simulink model "fuelcell"  (R2023a)
settings: Solver=VariableStepAuto  StartTime=0.0  StopTime=20  RelTol=1e-3
model workspace (MAT data in the model file):
  sweep1 = [0 5 10 15 20 25 30 35 40 45 50 55 60 65 70 75 80]
libraries: fl_lib x24, nesl_utility x12, ee_lib x2, spsCurrentVoltageSimscapeInterfaceLib x1, spsFuelCellStackLib x1, sps_lib x1
settings Model: Creator=connl  LastModifiedBy=connl

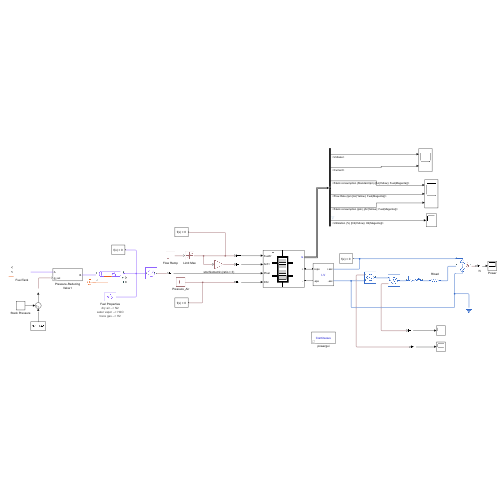
[thumbnail: Simulink's stored preview of the top-level diagram]
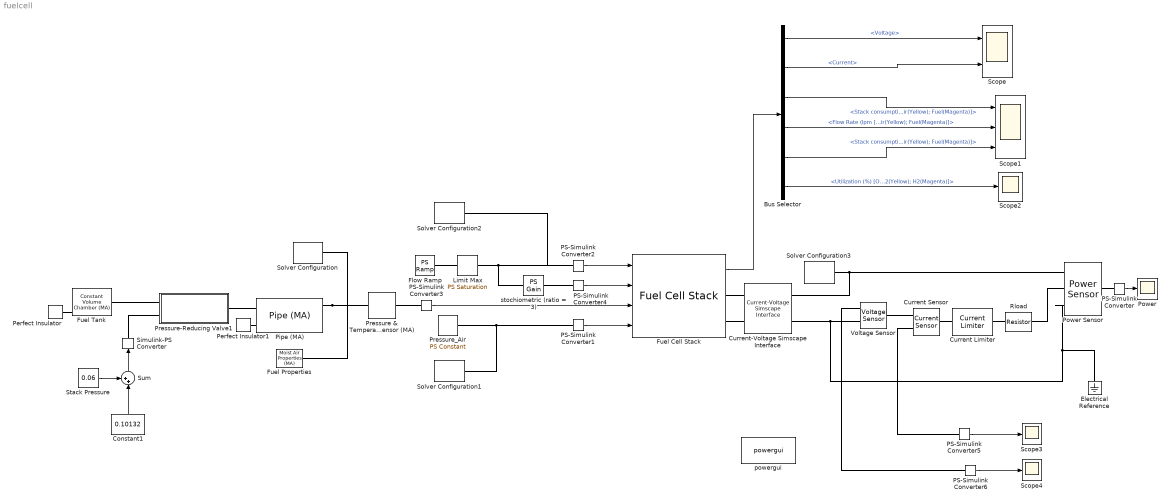
== system fuelcell ==
  Bus Selector : BusSelector  OutputSignals=Voltage,Current,Stack consumption (Standard lpm) [Air(Yellow); Fuel(Magenta)],Flow Rate (lpm [Air(Yellow); Fuel(Magenta)],Stack consumption (lpm) [Air(Yellow); Fuel(Magenta)],Utilization (%) [O2(Yellow); H2(Magenta)]
  Constant1 : Constant  Value=0.10132
  Current Limiter : ee_lib/Semiconductors & Converters/Current Limiter  iLim=80 A  vLim=0.1 V  gLim=1e-3 1/Ohm  thermal_mass=100 J/K  initial_temperature=298.15 K
      settings: InternalSimscapePortConfiguration="{\"Bottom\":[],\"Left\":[{\"id\":\"p\",\"label\":\"+\",\"type\":\"foundation.electrical.electrical\"}],\"Right\":[{\"id\":\"n\",\"label\":\"-\",\"type\":\"foundation.electrical.electrical\"}],\"Top\":[]}"
  Current Sensor : fl_lib/Electrical/Electrical Sensors/Current Sensor
  Current-Voltage Simscape Interface : spsCurrentVoltageSimscapeInterfaceLib/Current-Voltage Simscape Interface  DFT=off  FMode=Low pass filter (continuous)  T=1e-6  Ts=50e-6  i0=0  v0=0  Sd=Specialized Power Systems side  Measurements=off
      settings: LibrarySourceBlock=|
      | sps_lib/Utilities/Current-Voltage
      | Simscape Interface
  Electrical Reference : fl_lib/Electrical/Electrical Elements/Electrical Reference
  Flow Ramp : fl_lib/Physical Signals/Sources/PS Ramp  slope=1.667 lpm/s  start_time=0 s  initial_output=2 lpm
  Fuel Cell Stack : spsFuelCellStackLib/Fuel Cell Stack  PresetModel=PEMFC - 1.26 kW - 24 Vdc  FcType=0  Detailed=Detailed  Eoc=[42,35]  NomVI=[52,24.23]  EndVI=[100,20]  Nc=42  n=46  TOp=55  AirFr=2400  SuppPress=[1.5,1]  Comp=[99.95,21,1]  SignX=off  SignY=off  FlowRateH2=on  FlowRateAir=on  SystemTemp=off  SystemPH2=on  SystemPAir=on  FCDyn=off  FC_tau=1  Peak_O2=80  V_Under=10
      settings: LibrarySourceBlock=sps_lib/Sources/Fuel Cell Stack
  Fuel Properties : fl_lib/Moist Air/Utilities/Moist Air Properties (MA)  R_a=296.8 J/kg/K  T_TLU=[-56.55 -50 -40 -30 -20 -10 -5 -4 -3 -2 -1 0 1 2 3 4 5 10 20 30 40 50 60 70 80 90 100 110 120 130 140 150 160 170 180 190 200 210 220 230 240 250 260 270 280 290 300 310 320 330 340 350] degC  h_a_TLU=[224.312019475783 231.141016528663 241.564116974996 251.984329606098 262.402210767198 272.818266126753 278.025759131002 279.067222480148 280.108675169779 281.150117667373 282.191550440608 283.232973957487 284.274388686473 285.315795096618 286.357193657682 287.39858484026 288.439969115894 293.646803474573 304.06022922571 314.473742203777 324.887858161051 335.303123493654 345.720119003427 356.139461810715 366.561805672305 376.987839945795 387.418287430292 397.85390130103 408.295461341278 418.743769658649 429.199646054884 439.663923199077 450.137441734658 460.621045430963 471.115576471389 481.621870952319 492.140754650669 502.67303910305 513.219518026408 523.780964098585 534.358126107445 544.951726469054 555.562459108678 566.190987693008 576.837944197865 587.503927792527 598.189504019663 608.89520424844 619.621525377624 630.368929765337 641.137845362314 651.928666026144] kJ/kg  mu_a_TLU=[13.7948920665312 14.136718735151 14.6513506072199 15.1575394445859 15.6556177860831 16.1459023391225 16.3882166949119 16.4364580271216 16.484626183061 16.5327214469937 16.5807441017456 16.6286944287114 16.6765727078615 16.7243792177482 16.7721142355126 16.8197780368914 16.8673708962236 17.1042805670559 17.5729330929829 18.0349108462106 18.4904598524977 18.9398140034241 19.3831957199835 19.8208165930053 20.2528779961256 20.6795716689317 21.101080269236 21.5175778943589 21.9292305719283 22.3361967211248 22.7386275855675 23.1366676391963 23.5304549665897 23.9201216191847 24.3057939488592 24.6875929202991 25.0656344035241 25.4400294478834 25.8108845387614 26.178301838167 26.5423794103038 26.9032114331518 27.2608883970194 27.6154972909606 27.96712177789 28.315842359167 28.6617365293689 29.0048789219164 29.3453414461711 29.6831934165754 30.0185016743671 30.3513307023604] s*uPa  k_a_TLU=[19.6296532607374 20.1533289725195 20.9436243615696 21.7231523445233 22.492306313909 23.2514823266989 23.6274403302585 23.7023472871786 23.7771601872884 23.8518793809024 23.9265052168265 24.0010380423605 24.0754782033001 24.1498260439393 24.2240819070729 24.2982461339996 24.3723190645241 24.7413260601341 25.4726839899413 26.1954347636057 26.9098870600572 27.6163358040134 28.3150627088262 29.0063368423447 29.6904152006066 30.3675432785589 31.0379556302294 31.7018764131555 32.3595199136277 33.0110910505971 33.6567858570436 34.2967919382928 34.9312889072676 35.5604487970156 36.1844364511046 36.8034098926428 37.417520672793 38.0269141997105 38.63173004887 39.2321022557508 39.828159591842 40.4200258249072 41.0078199644172 41.591656493024 42.171645584909 42.7478933117983 43.3205018373934 43.8895696009277 44.4551914905138 45.0174590069098 45.5764604182929 46.1322809065919] mW/m/K  p_min=1 kPa  p_max=inf MPa  T_min=-56.55 degC  T_max=350 degC  properties_range_check=simscape.enum.assert.action.error  p_atm=0.101325 MPa  T_atm=20 degC  R_w=461.523 J/kg/K  p_ws_TLU=[1.71168953425982e-06; 3.93770601979424e-06; 1.28411717710344e-05; 3.80051394873809e-05; .00010323902900209; .000259873810798063; .000401741022116384; .000437454836117844; .000476040820618202; .000517704666185737; .000562664883741207; .000611212677444345; .000657088049117899; .000705987905898279; .000758082381149132; .000813549384183233; .000872574861129522; .00122818386934022; .0023392147667769; .00424668834054807; .00738442748706953; .0123512704340234; .0199458019246787; .0312006356960619; .0474147199263783; .0701823607447713; .10141797792131; .143375967241115; .198665399739302; .270259606559999; .361500961984849; .476101381081492; .618139196722055; .792053183687694; 1.0026345688121; 1.25501792086105; 1.55467186826983; 1.90739066433297; 2.31928772772542; 2.79679245576864; 3.34665187151016; 3.97593907083533; 4.69207105435535; 5.5028394740883; 6.41645928168037; 7.4416425436169; 8.58770832955728; 9.86474556030261; 11.2838558865497; 12.8575218898034; 14.6001810568052; 16.5291642526045] MPa  h_w_vap_TLU=[2836.88241275372; 2837.81392500514; 2838.63937175807; 2838.7309929628; 2838.06905313927; 2836.62597341095; 2835.60023952573; 2835.37006381376; 2835.13143158077; 2834.88429145066; 2834.62859062897; 2500.93420564316; 2498.55329907119; 2496.17495082036; 2493.79885912205; 2491.42474723191; 2489.05236104642; 2477.20875029194; 2453.54955988604; 2429.83856603313; 2406.00136954922; 2381.97406342174; 2357.69101156389; 2333.08088387814; 2308.06565480412; 2282.56034405021; 2256.47287422313; 2229.70428017508; 2202.14968030993; 2173.69998896199; 2144.24368406447; 2113.66758247452; 2081.85585110571; 2048.68725710494; 2014.03141249899; 1977.7449923284; 1939.66849592886; 1899.62342931686; 1857.40930169838; 1812.79975416601; 1765.53721731251; 1715.32525772152; 1661.81700477787; 1604.59703745016; 1543.1534616334; 1476.83692476464; 1404.80240352424; 1325.92091736114; 1238.61667822208; 1140.5102987018; 1027.62017777647; 892.733785613825] kJ/kg  h_w_TLU=[2396.55944251649; 2408.68643343608; 2427.1988031141; 2445.702165897; 2464.18429108356; 2482.62529466839; 2491.82135326629; 2493.6580151792; 2495.49372578218; 2497.32843835745; 2499.16210446923; 2500.99462758899; 2502.83092214066; 2504.6665223621; 2506.50140563013; 2508.335548891; 2510.16892865793; 2519.32352241995; 2537.56068088674; 2555.67742615292; 2573.6403223998; 2591.4109179101; 2608.9455037701; 2626.19492016262; 2643.10444358428; 2659.61377634497; 2675.58278696023; 2696.1846256545; 2716.49989553741; 2736.6235210957; 2756.61216047011; 2776.50561773853; 2796.33378922508; 2816.11979583049; 2835.88181423877; 2855.63430574511; 2875.38889327595; 2895.15500577172; 2914.94035964689; 2934.75132290228; 2954.59319330244; 2974.47041285505; 2994.38673458964; 3014.34535328009; 3034.34900867103; 3054.40006755764; 3074.50058946898; 3094.65237953784; 3114.85703128106; 3135.11596137801; 3155.43043805905; 3175.80160435813] kJ/kg  mu_w_TLU=[6.81365662228272; 7.04953750742707; 7.40970098298307; 7.76991278093907; 8.13017290129507; 8.49048134405107; 8.67065368632907; 8.70668960445667; 8.74272600580827; 8.77876289038387; 8.81480025818347; 8.85083810920707; 8.88687644345467; 8.92291526092627; 8.95895456162187; 8.99499434554147; 9.03103461268507; 9.21124319676307; 9.57169660671907; 9.93219833907507; 10.2927483938311; 10.6533467709871; 11.0139934705431; 11.3746884924991; 11.7354318368551; 12.0962235036111; 12.4570634927671; 12.8179518043231; 13.1788884382791; 13.5398733946351; 13.9009066733911; 14.2619882745471; 14.6231181981031; 14.9842964440591; 15.3455230124151; 15.7067979031711; 16.0681211163271; 16.4294926518831; 16.7909125098391; 17.1523806901951; 17.5138971929511; 17.8754620181071; 18.2370751656631; 18.5987366356191; 18.9604464279751; 19.3222045427311; 19.6840109798871; 20.0458657394431; 20.4077688213991; 20.7697202257551; 21.1317199525111; 21.4937680016671] s*uPa  k_w_TLU=[11.46288215976; 11.941997488935; 12.676358586935; 13.414208884935; 14.155548382935; 14.900377080935; 15.274099879935; 15.348949115735; 15.423833243535; 15.498752263335; 15.573706175135; 15.648694978935; 15.723718674735; 15.798777262535; 15.873870742335; 15.948999114135; 16.024162377935; 16.400502076935; 17.155798374935; 17.914583872935; 18.676858570935; 19.442622468935; 20.211875566935; 20.984617864935; 21.760849362935; 22.540570060935; 23.323779958935; 24.110479056935; 24.900667354935; 25.694344852935; 26.491511550935; 27.292167448935; 28.096312546935; 28.903946844935; 29.715070342935; 30.529683040935; 31.347784938935; 32.169376036935; 32.994456334935; 33.823025832935; 34.655084530935; 35.490632428935; 36.329669526935; 37.172195824935; 38.018211322935; 38.867716020935; 39.720709918935; 40.577193016935; 41.437165314935; 42.300626812935; 43.167577510935; 44.038017408935] mW/m/K  D_w=25 mm^2/s  trace_gas_model=foundation.enum.trace_gas_model.track_properties  R_g=4124.48151675695 J/kg/K  h_g_TLU=[2783.66044045879 2873.94181645932 3012.62601981068 3152.22537301871 3292.62486344326 3433.7213835968 3504.50184295996 3518.67512520997 3532.85394543712 3547.03822323045 3561.22787913325 3575.42283463482 3589.62301216223 3603.82833507219 3618.0387276429 3632.25411506595 3646.4744234383 3717.64725530348 3860.3219873489 4003.3828816304 4146.77354613486 4290.44463593559 4434.35318483605 4578.46197843019 4722.7389683309 4867.15672726297 5011.69194456718 5156.32496143709 5301.03934494342 5445.82149962224 5590.6603151415 5735.54684833147 5880.47403768083 6025.43644826542 6170.4300449914 6315.45199199528 6460.50047604533 6605.57455182556 6750.67400704912 6895.79924543541 7040.95118568927 7186.1311747363 7331.34091359044 7476.58239435534 7621.85784698693 7767.16969456766 7912.52051596217 8057.91301483815 8203.34999414341 8348.83433523064 8494.36898091475 8639.95692183309] kJ/kg  mu_g_TLU=[7.13280985169147 7.28192581803172 7.50683010986396 7.72860158311813 7.94743907374985 8.16352107178216 8.27057966039486 8.29191522386247 8.31322574339419 8.33451136221049 8.35577222214406 8.37700846365822 8.39822022586488 8.41940764654233 8.44057086215268 8.461710007859 8.48282521754219 8.58804682376172 8.79676834158601 9.00329345223078 9.2077322236417 9.41018554308578 9.61074613691738 9.809499451117 10.0065244149257 10.2018941058184 10.3956763308132 10.5879341365094 10.7787262581519 10.9681075163184 11.156129168438 11.342839221216 11.5282827091027 11.7125019431712 11.8955367341236 12.0774245926121 12.2582009096067 12.4378991191677 12.6165508456572 12.7941860371557 12.9708330866186 13.1465189421111 13.3212692072909 13.4951082331655 13.6680592020247 13.8401442043429 14.011384309352 14.1817996299056 14.3514093821846 14.520231940734 14.6882848892642 14.8555850676093] s*uPa  k_g_TLU=[142.834673487453 146.602208511061 152.236222042957 157.732550941948 163.097652939664 168.338595936873 170.914793442425 171.426608923333 171.937300226766 172.446874689218 172.955339634979 173.462702374715 173.968970204106 174.47415040255 174.978250231913 175.48127693535 175.983237736166 178.477304495221 183.389581255575 188.206454189023 192.934525090876 197.580042887656 202.14889050071 206.646585109232 211.078287130673 215.448814629342 219.762660868078 224.024013435935 228.236773894856 232.404577248187 236.530810785993 240.61863203742 244.670985680918 248.690619345047 252.680098287219 256.641818973249 260.57802160272 264.4908016382 268.38212040295 272.253814814231 276.107606318911 279.945109095949 283.767837587053 287.577213413001 291.374571728986 295.161167068166 298.938178718576 302.706715674597 306.467821200562 310.222477040649 313.971607306067 317.716082067666] mW/m/K  D_g=74 mm^2/s
      settings: AttributesFormatString=|
      | dry air --> N2
      | water vapor --> H2O
      | trace gas --> H2
  Fuel Tank : fl_lib/Moist Air/Elements/Constant Volume Chamber (MA)  volume=7 l  num_ports=foundation.enum.num_ports.one  area_A=7.854e-5 m^2  area_B=0.01 m^2  area_C=0.01 m^2  area_D=0.01 m^2  RH_ws=1  time_constant=1e-3 s  moisture_trace_gas_source=foundation.enum.moisture_trace_gas_source.none  moisture_source_spec=foundation.enum.moisture_source_spec.vapor  moisture_mass_flow=0 kg/s  moisture_temperature_spec=foundation.enum.temperature_spec.atmospheric  moisture_temperature=293.15 K  trace_gas_mass_flow=0 kg/s  trace_gas_temperature_spec=foundation.enum.temperature_spec.atmospheric  trace_gas_temperature=293.15 K  p_I_specify=on  p_I_priority=High  p_I=350 bar  p_I_nominal_specify=off  p_I_nominal_unit=MPa  p_I_nominal_value=1  T_I_specify=on  T_I_priority=High  T_I=20 degC  T_I_nominal_specify=off  T_I_nominal_unit=K  T_I_nominal_value=1  RH_I_specify=off  RH_I_priority=High  RH_I=0  RH_I_nominal_specify=off  RH_I_nominal_unit=1  RH_I_nominal_value=1  x_w_I_specify=off  x_w_I_priority=None  x_w_I=0  x_w_I_nominal_specify=off  x_w_I_nominal_unit=1  x_w_I_nominal_value=1  y_w_I_specify=off  y_w_I_priority=None  y_w_I=0  y_w_I_nominal_specify=off  y_w_I_nominal_unit=1  y_w_I_nominal_value=1  HR_I_specify=off  HR_I_priority=None  HR_I=0  HR_I_nominal_specify=off  HR_I_nominal_unit=1  HR_I_nominal_value=1  x_g_I_specify=on  x_g_I_priority=None  x_g_I=0  x_g_I_nominal_specify=off  x_g_I_nominal_unit=1  x_g_I_nominal_value=1  y_g_I_specify=on  y_g_I_priority=High  y_g_I=0.9997  y_g_I_nominal_specify=off  y_g_I_nominal_unit=1  y_g_I_nominal_value=1
      settings: InternalSimscapePortConfiguration="{\"Bottom\":[],\"Left\":[{\"id\":\"A\",\"label\":\"A\",\"type\":\"foundation.moist_air.moist_air\"}],\"Right\":[{\"id\":\"W\",\"label\":\"W\",\"type\":\"output\"},{\"id\":\"F\",\"label\":\"F\",\"type\":\"output\"},{\"id\":\"H\",\"label\":\"H\",\"type\":\"foundation.thermal.thermal\"}],\"Top\":[]}"
  Limit Max : fl_lib/Physical Signals/Nonlinear Operators/PS Saturation  upper_limit=100 lpm  lower_limit=0 lpm
  PS-Simulink Converter : nesl_utility/PS-Simulink Converter  PhysicalDomain=network_engine_domain  SubClassName=ps_output  LeftPortType=input  RightPortType=output  PseudoPeriodic=off  Frequencies=[]  VectorFormat=1-D array  Unit=W  AffineConversion=off
  PS-Simulink Converter{1..6} (6 alike) : nesl_utility/PS-Simulink Converter  PhysicalDomain=network_engine_domain  SubClassName=ps_output  LeftPortType=input  RightPortType=output  PseudoPeriodic=off  Frequencies=[]  VectorFormat=inherit  Unit=inherit  AffineConversion=off
  Perfect Insulator : fl_lib/Thermal/Thermal Elements/Perfect Insulator  T_specify=off  T_priority=None  T=0 K  T_nominal_specify=off  T_nominal_unit=K  T_nominal_value=1
  Perfect Insulator1 : fl_lib/Thermal/Thermal Elements/Perfect Insulator  T_specify=off  T_priority=None  T=0 K  T_nominal_specify=off  T_nominal_unit=K  T_nominal_value=1
  Pipe (MA) : fl_lib/Moist Air/Elements/Pipe (MA)  length=1 m  area=7.854e-5 m^2  Dh=0.01 m  length_add=0.1 m  roughness=15e-6 m  Re_lam=2000  Re_tur=4000  shape_factor=64  Nu_lam=3.66  wall_condensation=simscape.enum.onoff.off  RH_ws=1  time_constant=1e-3 s  moisture_trace_gas_source=foundation.enum.moisture_trace_gas_source.none  moisture_source_spec=foundation.enum.moisture_source_spec.vapor  moisture_mass_flow=0 kg/s  moisture_temperature_spec=foundation.enum.temperature_spec.atmospheric  moisture_temperature=293.15 K  trace_gas_mass_flow=0 kg/s  trace_gas_temperature_spec=foundation.enum.temperature_spec.atmospheric  trace_gas_temperature=293.15 K  p_I_specify=on  p_I_priority=High  p_I=0.10132 MPa  p_I_nominal_specify=off  p_I_nominal_unit=MPa  p_I_nominal_value=1  T_I_specify=on  T_I_priority=High  T_I=20 degC  T_I_nominal_specify=off  T_I_nominal_unit=K  T_I_nominal_value=1  RH_I_specify=off  RH_I_priority=High  RH_I=0  RH_I_nominal_specify=off  RH_I_nominal_unit=1  RH_I_nominal_value=1  x_w_I_specify=off  x_w_I_priority=None  x_w_I=0  x_w_I_nominal_specify=off  x_w_I_nominal_unit=1  x_w_I_nominal_value=1  y_w_I_specify=off  y_w_I_priority=None  y_w_I=0  y_w_I_nominal_specify=off  y_w_I_nominal_unit=1  y_w_I_nominal_value=1  HR_I_specify=off  HR_I_priority=None  HR_I=0  HR_I_nominal_specify=off  HR_I_nominal_unit=1  HR_I_nominal_value=1  x_g_I_specify=on  x_g_I_priority=None  x_g_I=0  x_g_I_nominal_specify=off  x_g_I_nominal_unit=1  x_g_I_nominal_value=1  y_g_I_specify=on  y_g_I_priority=High  y_g_I=0.9997  y_g_I_nominal_specify=off  y_g_I_nominal_unit=1  y_g_I_nominal_value=1
  Power : Scope
  Power Sensor : ee_lib/Sensors & Transducers/Power Sensor  measurement_type=1  averaging_period=1e-4 s
  Pressure & Temperature Sensor (MA) : fl_lib/Moist Air/Sensors/Pressure & Temperature Sensor (MA)  reference=foundation.enum.MeasurementReference.absolute  pressure=true  pressure_spec=foundation.enum.PressureMeasementSpec.Absolute  temperature=false
      settings: InternalSimscapePortConfiguration="{\"Bottom\":[],\"Left\":[{\"id\":\"A\",\"label\":\"A\",\"type\":\"foundation.moist_air.moist_air\"}],\"Right\":[{\"id\":\"Pa\",\"label\":\"Pa\",\"type\":\"output\"}],\"Top\":[]}"
  Pressure-Reducing Valve1 : Subsystem  Tag=PublishSubsystem  mask(Pressure-Reducing Valve){D=0.01, r_min=1e-4, r_max=0.2, p_range=0.005}
      mask prompts: D "Connecting tube diameter (m)"; r_min "Min diameter ratio"; r_max "Max diameter ratio"; p_range "Pressure regulation range (MPa)"
      mask help: This subsystem models a pressure reducing valve that maintains a set pressure at port B. The valve is normally open. When the pressure is above the set pressure, it is fully closed.
  Pressure_Air : fl_lib/Physical Signals/Sources/PS Constant  constant=1 bar
  Rload : fl_lib/Electrical/Electrical Elements/Resistor  R=1 Ohm  i_specify=off  i_priority=None  i=0 A  i_nominal_specify=off  i_nominal_unit=A  i_nominal_value=1  v_specify=off  v_priority=None  v=0 V  v_nominal_specify=off  v_nominal_unit=V  v_nominal_value=1
  Scope : Scope  NumInputPorts=2
  Scope1 : Scope  NumInputPorts=3
  Scope2 : Scope
  Scope3 : Scope
  Scope4 : Scope
  Simulink-PS Converter : nesl_utility/Simulink-PS Converter  PhysicalDomain=network_engine_domain  SubClassName=ps_input  LeftPortType=input  RightPortType=output  PseudoPeriodic=off  Frequencies=[]  NoiseDistribution=none  NoiseParameters=[]  Unit=MPa  AffineConversion=off  FilteringAndDerivatives=provide  SimscapeFilterOrder=1  InputFilterTimeConstant=0.001  UdotUserProvided=0
  Solver Configuration{,1..3} (4 alike) : nesl_utility/Solver Configuration  PhysicalDomain=network_engine_domain  SubClassName=solver  LeftPortType=input  RightPortType=generic  Tones=[]  Harmonics=[]  SimulateNoise=off  Profile=off  UseLocalSampling=off  EnableSwitchedLinearOptims=on  FrequencyDomain=off  UseCCode=off  RelTol=0.001  AbsTol=0.001  MinStep=1e-09  ToWorkspace=off  RevertToSquareIcSolve=off  NumHomotopyIterations=100  PhasorMode=off  PhasorModeNumHarmonics=1  ConsistencySolver=NEWTON_XTOL_AFTER_FTOL  IndexReductionMethod=DerivativeReplacement  DoDC=off  ResidualTolerance=1e-09  ConsistencyTolSource=GLOBAL  ConsistencyAbsTol=0.001  ConsistencyRelTol=0.001  ConsistencyTolFactor=0.001  UseLocalSolver=off  LocalSolverChoice=NE_BACKWARD_EULER_ADVANCER  ResolveIndetEquations=on  FunctionEvalNumThread=1  LocalSolverSampleTime=0.001  DoFixedCost=off  MaxNonlinIter=3  MaxModeIter=2  ComputeImpulses=off  ImpulseIterations=2  LinearAlgebra=auto  LinearAlgebraNumThread=0  EquationFormulation=NE_TIME_EF  DelaysMemoryBudget=1024  AutomaticFiltering=on  FilteringTimeConstant=0.001  PartitionStorageMethod=AS_NEEDED  PartitionMemoryBudget=1024  PartitionMethod=ROBUST
  Stack Pressure : Constant  Value=0.06
  Sum : Sum  Inputs=++|
  Voltage Sensor : fl_lib/Electrical/Electrical Sensors/Voltage Sensor
  powergui : sps_lib/powergui  Priority=1  SimulationMode=Continuous  SampleTime=50e-6  frequency=60  Iterations=50  frequencyindice=0  Pbase=100e6  ErrMax=1e-4  UnitsV=kV  UnitsW=MW  buscounter=0  FunctionMessages=off  echomessages=off  EnableUseOfTLC=off  CurrentSourceSwitches=off  DisableSnubberDevices=off  DisableRonSwitches=off  DisableVfSwitches=off  DisplayEquations=off  AutomaticDiscreteSolvers=off  SolverType=Tustin/Backward Euler (TBE)  Interpol=off  ExternalGateDelay=off  methode=off  Ts=100  x0status=blocks  SPID=on  SwTol=0  HookPort=off  NonlinearTolerance=1e-4  nMaxIteration=100  ContinueOnMaxIteration=off  RestoreLinks=warning  ResistiveCurrentMeasurement=off  Frange=[0:2:500]  Ylog=off  Xlog=on  ShowGrid=off  save=off  variable=ZData  structure=0  ZoomFFT=off  StartTime=0.0  cycles=1  DisplayStyle=1  fundamental=60  FreqAxis=off  MaxFrequency=1000  frequencyindicesteady=1  RmsSteady=1  display=off
  stochiometric (ratio = 3) : fl_lib/Physical Signals/Functions/PS Gain  gain=3.0
  wires:
  Stack Pressure/1 -> Sum/1
  Constant1/1 -> Sum/2
  PS-Simulink Converter/1 -> Power/1
  Sum/1 -> Simulink-PS Converter/1
  PS-Simulink Converter1/1 -> Fuel Cell Stack/4
  PS-Simulink Converter4/1 -> Fuel Cell Stack/2
  PS-Simulink Converter2/1 -> Fuel Cell Stack/1
  PS-Simulink Converter3/1 -> Fuel Cell Stack/3
  Fuel Cell Stack/1 -> Bus Selector/1
  Bus Selector/2 -> Scope/2  "<Current>"
  Bus Selector/4 -> Scope1/2  "<Flow Rate (lpm [Air(Yellow); Fuel(Magenta)]>"
  Bus Selector/5 -> Scope1/3  "<Stack consumption (lpm) [Air(Yellow); Fuel(Magenta)]>"
  Bus Selector/1 -> Scope/1  "<Voltage>"
  Bus Selector/3 -> Scope1/1  "<Stack consumption (Standard lpm) [Air(Yellow); Fuel(Magenta)]>"
  Bus Selector/6 -> Scope2/1  "<Utilization (%) [O2(Yellow); H2(Magenta)]>"
  PS-Simulink Converter5/1 -> Scope3/1
  PS-Simulink Converter6/1 -> Scope4/1
  connections:
  Power Sensor/LConn1 -- Solver Configuration3/RConn1 -- Current-Voltage Simscape Interface/RConn1
  stochiometric (ratio = 3)/LConn1 -- Solver Configuration2/RConn1 -- PS-Simulink Converter2/LConn1 -- Limit Max/RConn1
  Pipe (MA)/RConn1 -- Solver Configuration/RConn1 -- Pressure & Temperature Sensor (MA)/LConn1 -- Fuel Properties/RConn1
  Pipe (MA)/LConn1 -- Pressure-Reducing Valve1/RConn1
  Perfect Insulator1/LConn1 -- Pipe (MA)/LConn2
  Perfect Insulator/LConn1 -- Fuel Tank/RConn3
  Pressure-Reducing Valve1/LConn2 -- Simulink-PS Converter/RConn1
  Power Sensor/RConn1 -- PS-Simulink Converter/LConn1
  Limit Max/LConn1 -- Flow Ramp/RConn1
  Pressure_Air/RConn1 -- Solver Configuration1/RConn1 -- PS-Simulink Converter1/LConn1
  PS-Simulink Converter4/LConn1 -- stochiometric (ratio = 3)/RConn1
  PS-Simulink Converter3/LConn1 -- Pressure & Temperature Sensor (MA)/RConn1
  Pressure-Reducing Valve1/LConn1 -- Fuel Tank/LConn1
  Current-Voltage Simscape Interface/LConn1 -- Fuel Cell Stack/RConn1
  Fuel Cell Stack/RConn2 -- Current-Voltage Simscape Interface/LConn2
  Power Sensor/LConn3 -- Electrical Reference/LConn1 -- Current-Voltage Simscape Interface/RConn2 -- Voltage Sensor/RConn2
  Current Sensor/RConn1 -- PS-Simulink Converter5/LConn1
  Current Limiter/RConn1 -- Current Sensor/LConn1
  Voltage Sensor/LConn1 -- Current Sensor/RConn2
  Voltage Sensor/RConn1 -- PS-Simulink Converter6/LConn1
  Power Sensor/LConn2 -- Rload/LConn1
  Rload/RConn1 -- Current Limiter/LConn1

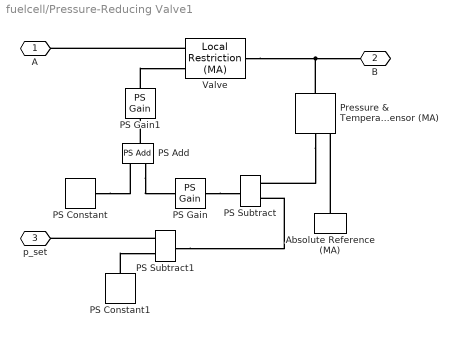
== system fuelcell/Pressure-Reducing Valve1 ==
  Absolute Reference (MA) : fl_lib/Moist Air/Elements/Absolute Reference (MA)
  PS Add : fl_lib/Physical Signals/Functions/PS Add
  PS Constant : fl_lib/Physical Signals/Sources/PS Constant  constant=r_max^2
  PS Constant1 : fl_lib/Physical Signals/Sources/PS Constant  constant=p_range MPa
  PS Gain : fl_lib/Physical Signals/Functions/PS Gain  gain=(r_min^2 - r_max^2)/p_range 1/MPa
  PS Gain1 : fl_lib/Physical Signals/Functions/PS Gain  gain=pi*D^2/4 m^2
  PS Subtract : fl_lib/Physical Signals/Functions/PS Subtract
  PS Subtract1 : fl_lib/Physical Signals/Functions/PS Subtract
  Pressure & Temperature Sensor (MA) : fl_lib/Moist Air/Sensors/Pressure & Temperature Sensor (MA)  reference=foundation.enum.MeasurementReference.difference  pressure=true  pressure_spec=foundation.enum.PressureMeasementSpec.Absolute  temperature=true
      settings: InternalSimscapePortConfiguration="{\"Bottom\":[{\"id\":\"T\",\"label\":\"T\",\"type\":\"output\"}],\"Left\":[{\"id\":\"A\",\"label\":\"A\",\"type\":\"foundation.moist_air.moist_air\"}],\"Right\":[{\"id\":\"B\",\"label\":\"B\",\"type\":\"foundation.moist_air.moist_air\"},{\"id\":\"P\",\"label\":\"P\",\"type\":\"output\"}],\"Top\":[]}"
  Valve : fl_lib/Moist Air/Elements/Local Restriction (MA)  restriction_type=foundation.enum.restriction_type.variable  restriction_area=0.001 m^2  min_area=pi*(r_min*D)^2/4 m^2  max_area=pi*(r_max*D)^2/4 m^2  area=pi*D^2/4 m^2  Cd=0.64  B_lam=0.999
  A : PMIOPort  Side=Left
  B : PMIOPort  Port=2  Side=Right
  p_set : PMIOPort  Port=3  Side=Left
  connections:
  PS Constant1/RConn1 -- PS Subtract1/LConn2
  PS Subtract1/LConn1 -- p_set/RConn1
  PS Subtract1/RConn1 -- PS Subtract/LConn2
  PS Constant/RConn1 -- PS Add/LConn1
  PS Add/LConn2 -- PS Gain/RConn1
  PS Add/RConn1 -- PS Gain1/LConn1
  PS Gain/LConn1 -- PS Subtract/RConn1
  Pressure & Temperature Sensor (MA)/RConn2 -- PS Subtract/LConn1
  PS Gain1/RConn1 -- Valve/LConn2
  Absolute Reference (MA)/LConn1 -- Pressure & Temperature Sensor (MA)/RConn1
  Pressure & Temperature Sensor (MA)/LConn1 -- B/RConn1 -- Valve/RConn1
  Valve/LConn1 -- A/RConn1
